simulink model "KF"  (R2019a)
settings: Solver=VariableStepAuto  StartTime=0.0  StopTime=200  RelTol=1e-3
values from neighbouring files (symbols this model uses):
  g = 9.81    [Q2.m]
  k_d_phi = (2*zeta_phi*omega_n_phi-a_phi_1)/a_phi_2    [Q2.m]
  k_i_chi = omega_n_chi^2*V_g/g    [Q2.m]
  k_i_phi = 0    [Q2.m]
  k_p_chi = 2*zeta_chi*omega_n_chi*V_g/g    [Q2.m]
  k_p_phi = delta_a_max/e_phi_max*sign(a_phi_2)    [Q2.m]
  V_g = 580/3.6    (= 161.111111111)    [Q2.m]
undefined symbols (not defined in the file or in its folder): sigbuilder_block
libraries: simulink_extras x3
settings Model: Creator=Shuyuan  LastModifiedBy=zhy
settings DataIOCC: ReturnWorkspaceOutputs=off
settings DebuggingCC: PregeneratedLibrarySubsystemCodeDiagnostic=none  ArithmeticOperatorsInVariantConditions=warning
settings SFSimCC: SimUseLocalCustomCode=off
settings RTWCC: RTWUseLocalCustomCode=off

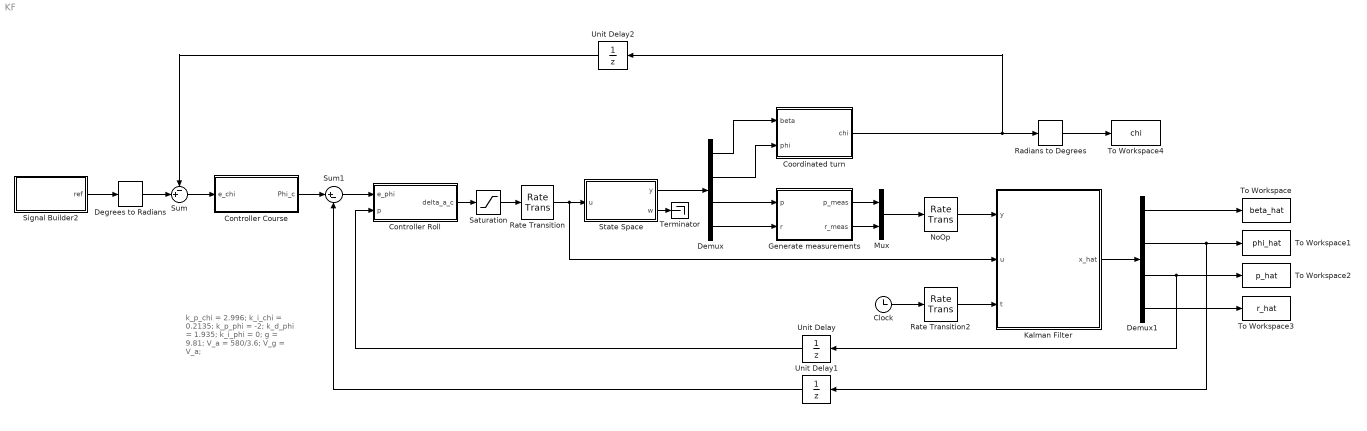
== system KF ==
  note: k_p_chi = 2.996;
      | k_i_chi = 0.2135;
      | k_p_phi = -2;
      | k_d_phi = 1.935;
      | k_i_phi = 0;
      |
      | g = 9.81;
      | V_a = 580/3.6;
      | V_g = V_a;
  Clock : Clock
  Controller Course : Subsystem
  Controller Roll : Subsystem
  Coordinated turn : Subsystem
  Degrees to Radians : simulink_extras/Transformations/Degrees to Radians
  Demux : Demux
  Demux1 : Demux
  Generate measurements : Subsystem
  Kalman Filter : MATLAB Function  TreatAsAtomicUnit=on
  Mux : Mux  Inputs=2
  NoOp : RateTransition
  Radians to Degrees : simulink_extras/Transformations/Radians to Degrees
  Rate Transition : RateTransition
  Rate Transition2 : RateTransition
  Saturation : Saturate  UpperLimit=30/180*pi  LowerLimit=-30/180*pi
  Signal Builder2 : Subsystem  Tag=STV Subsys  LoadFcn=sigbuilder_block('load');  StartFcn=sigbuilder_block('start');  StopFcn=sigbuilder_block('stop');  ClipboardFcn=sigbuilder_block('clipboard');  mask(Sigbuilder block){tuvar=[0:10]}
      mask help: Simulink:masks:SigbuilderBlock_MD
      mask init:
      | if ~strcmp(get_param(bdroot(gcbh),'SimulationStatus'),'stopped') tuvar = sigbuilder_block('maskInit'); end
      settings: CopyFcn=sigbuilder_block('copy');  DeleteFcn=sigbuilder_block('delete');  ModelCloseFcn=sigbuilder_block('modelClose');  PreSaveFcn=sigbuilder_block('preSave');  PauseFcn=sigbuilder_block('pause');  ContinueFcn=sigbuilder_block('continue');  NameChangeFcn=sigbuilder_block('namechange');  OpenFcn=sigbuilder_block('open',[411 163.2 550.8 400.2 ]);  CloseFcn=sigbuilder_block('close');
      mask Display: plot(0, 0, 100, 100,[2, 2, 32, 32, 2], [68, 8, 8, 68, 68],[32, 2], [38, 38], [32, 19, 2],[53, 60, 44], [32, 17, 17, 2],[16, 16, 31, 31]);txt = getActiveGroup(gcbh);text(2, 100, txt,'verticalAlignment', 'top');
  State Space : MATLAB Function  TreatAsAtomicUnit=on
  Sum : Sum  Inputs=-+|
  Sum1 : Sum  Inputs=|+-
  Terminator : Terminator
  To Workspace : ToWorkspace  VariableName=beta_hat  SaveFormat=Timeseries  SampleTime=-1
  To Workspace1 : ToWorkspace  VariableName=phi_hat  SaveFormat=Timeseries  SampleTime=-1
  To Workspace2 : ToWorkspace  VariableName=p_hat  SaveFormat=Timeseries  SampleTime=-1
  To Workspace3 : ToWorkspace  VariableName=r_hat  SaveFormat=Timeseries  SampleTime=-1
  To Workspace4 : ToWorkspace  VariableName=chi  SaveFormat=Timeseries  SampleTime=-1
  Unit Delay : UnitDelay  SampleTime=-1  HasFrameUpgradeWarning=on
  Unit Delay1 : UnitDelay  SampleTime=-1  HasFrameUpgradeWarning=on
  Unit Delay2 : UnitDelay  SampleTime=-1  HasFrameUpgradeWarning=on
  wires:
  Signal Builder2/1(ref) -> Degrees to Radians/1
  Sum/1 -> Controller Course/1(e_chi)
  Controller Course/1(Phi_c) -> Sum1/1
  Sum1/1 -> Controller Roll/1(e_phi)
  Controller Roll/1(delta_a_c) -> Saturation/1
  Rate Transition/1 -> Kalman Filter/2(u), State Space/1(u)
  State Space/1(y) -> Demux/1
  Demux/1 -> Coordinated turn/1(beta)
  Demux/2 -> Coordinated turn/2(phi)
  Demux/3 -> Generate measurements/1(p)
  Demux/4 -> Generate measurements/2(r)
  Clock/1 -> Rate Transition2/1
  Rate Transition2/1 -> Kalman Filter/3(t)
  Demux1/1 -> To Workspace/1
  Demux1/3 -> Unit Delay/1, To Workspace2/1
  Demux1/2 -> Unit Delay1/1, To Workspace1/1
  Demux1/4 -> To Workspace3/1
  Unit Delay/1 -> Controller Roll/2(p)
  Unit Delay1/1 -> Sum1/2
  State Space/2(w) -> Terminator/1
  Generate measurements/2(r_meas) -> Mux/2
  Generate measurements/1(p_meas) -> Mux/1
  Mux/1 -> NoOp/1
  NoOp/1 -> Kalman Filter/1(y)
  Kalman Filter/1(x_hat) -> Demux1/1
  Saturation/1 -> Rate Transition/1
  Radians to Degrees/1 -> To Workspace4/1
  Coordinated turn/1(chi) -> Unit Delay2/1, Radians to Degrees/1
  Degrees to Radians/1 -> Sum/2
  Unit Delay2/1 -> Sum/1

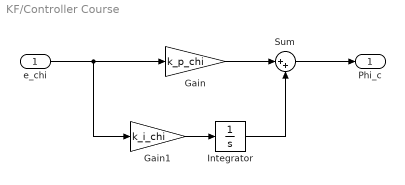
== system KF/Controller Course ==
  e_chi : Inport
  Gain : Gain  Gain=k_p_chi
  Gain1 : Gain  Gain=k_i_chi
  Integrator : Integrator
  Sum : Sum  Inputs=|++
  Phi_c : Outport
  wires:
  Sum/1 -> Phi_c/1
  Gain/1 -> Sum/1
  e_chi/1 -> Gain1/1, Gain/1
  Gain1/1 -> Integrator/1
  Integrator/1 -> Sum/2

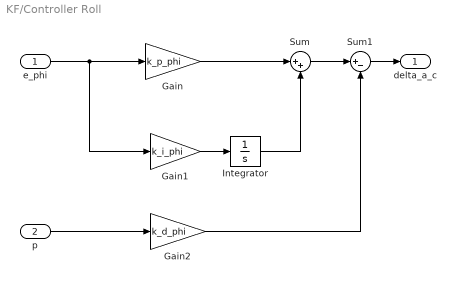
== system KF/Controller Roll ==
  e_phi : Inport
  p : Inport  Port=2
  Gain : Gain  Gain=k_p_phi
  Gain1 : Gain  Gain=k_i_phi
  Gain2 : Gain  Gain=k_d_phi
  Integrator : Integrator
  Sum : Sum  Inputs=|++
  Sum1 : Sum  Inputs=|+-
  delta_a_c : Outport
  wires:
  Gain/1 -> Sum/1
  e_phi/1 -> Gain1/1, Gain/1
  Gain1/1 -> Integrator/1
  Integrator/1 -> Sum/2
  Sum/1 -> Sum1/1
  Sum1/1 -> delta_a_c/1
  p/1 -> Gain2/1
  Gain2/1 -> Sum1/2

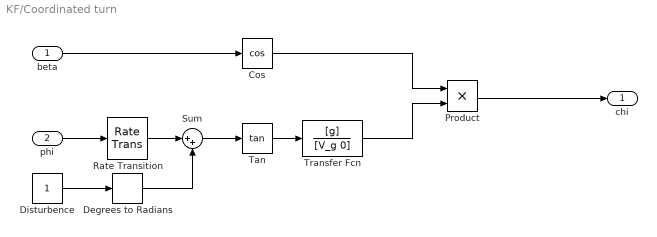
== system KF/Coordinated turn ==
  beta : Inport
  phi : Inport  Port=2
  Cos : Trigonometry  Operator=cos
  Degrees to Radians : simulink_extras/Transformations/Degrees to Radians
  Disturbence : Constant
  Product : Product
  Rate Transition : RateTransition
  Sum : Sum  Inputs=|++
  Tan : Trigonometry  Operator=tan
  Transfer Fcn : TransferFcn  Numerator=[g]  Denominator=[V_g 0]
  chi : Outport
  wires:
  phi/1 -> Rate Transition/1
  Disturbence/1 -> Degrees to Radians/1
  beta/1 -> Cos/1
  Sum/1 -> Tan/1
  Tan/1 -> Transfer Fcn/1
  Cos/1 -> Product/1
  Transfer Fcn/1 -> Product/2
  Degrees to Radians/1 -> Sum/2
  Rate Transition/1 -> Sum/1
  Product/1 -> chi/1

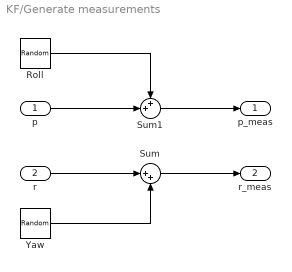
== system KF/Generate measurements ==
  p : Inport
  r : Inport  Port=2
  Roll : RandomNumber  Variance=(0.2*pi/180)^2  SampleTime=0.01
  Sum : Sum  Inputs=|++
  Sum1 : Sum  Inputs=++|
  Yaw : RandomNumber  Variance=(0.2*pi/180)^2  SampleTime=0.01
  p_meas : Outport
  r_meas : Outport  Port=2
  wires:
  p/1 -> Sum1/2
  Sum1/1 -> p_meas/1
  r/1 -> Sum/1
  Sum/1 -> r_meas/1
  Yaw/1 -> Sum/2
  Roll/1 -> Sum1/1

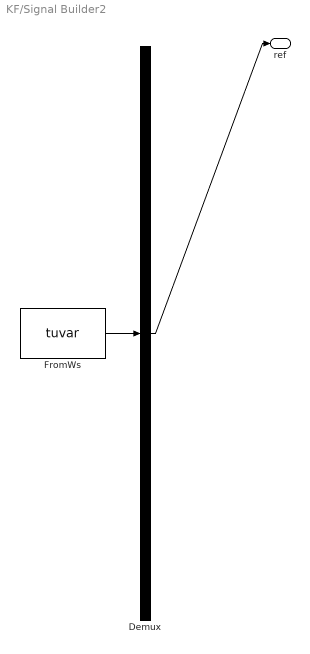
== system KF/Signal Builder2 ==
  Demux : Demux  Tag=STV Demux  Outputs=1
  FromWs : FromWorkspace  Tag=STV FromWs  VariableName=tuvar  SampleTime=0
      SigBuilderData=|
      | common.afterFinalStr = 'Extrapolate'
      | common.sampleTime = 0
      | dataSet.timeRange = [0 200]
      | dataSet.name = 'Group 1'
      | sbobj.Groups.Name = 'Group 1'
      | sbobj.Groups.Signals.Name = 'ref'
      | sbobj.Groups.Signals.XData = [0 25 25 75 75 125 125 200]
      | sbobj.Groups.Signals.YData = [0 0 5 5 10 10 15 15]
      | sbobj.Groups.TimeRange = [0 200]
  ref : Outport  Tag=STV Outport
  wires:
  FromWs/1 -> Demux/1
  Demux/1 -> ref/1

== matlab function KF/Kalman Filter ==
  settings: updateMethod=DISCRETE  sampleTime=0.01
  data: y input; x_hat output; u input; t input
function x_hat = Kalman_filter(y,u,t)

persistent xhat;
persistent xbar;
persistent P;

%% KF parameters
h = 0.01;
A_k = [-0.322, 0.052, 0.028, -1.12;
       0, 0, 1, -0.001;   
       -10.6, 0, -2.87, 0.46;
       6.87, 0, -0.04, -0.32];
B_k = [0.002; 0; -0.65; -0.02];
C_k = [0, 0, 1, 0;
       0, 0, 0, 1];
E_k = eye(4);
I = eye(4);
A_d = I+h*A_k;
B_d = h*B_k;
E_d = E_k;
Q = h*10^(-6)*diag([0.001,1,100,10]);
r = (0.2*pi/360)^2;
R = diag([r,r]);

%% Initial conditions
if isempty(xbar)
    xbar = [0;0;0;0];
    P = [0, 0, 0, 0;
         0, 0, 0, 0;
         0, 0, 0, 0;
         0, 0, 0, 0];
end

%% KF calculation
% if t <= 100
%     if mod(t, h) == 0
%     z = y;
%     H = C_k;
%     else
%     z = [0;0];
%     H = [0, 0, 0, 0; 0, 0, 0, 0];
%     end
% else
%     z = [0;0];
%     H = [0, 0, 0, 0; 0, 0, 0, 0];
% end


 if mod(t, h) == 0
    z = y;
    H = C_k;
 else
    z = [0;0];
    H = [0, 0, 0, 0; 0, 0, 0, 0];
 end



K = P*H'/(H*P*H'+R);
xhat = xbar+K*(z-H*xbar);
P = (I-K*H)*P*(I-K*H)'+K*R*K';

xbar = A_d*xhat+B_d*u;
P = A_d*P*A_d'+E_d*Q*E_d';

%% States output
x_hat = xhat;

== matlab function KF/State Space ==
  settings: updateMethod=DISCRETE  sampleTime=0.01
  data: u input; y output; w output
function [y,w] = state_space(u)
% Generate the output of the state space

    % Persistent variables to be kept between function calls
    persistent counter; % Variable for checking if it is the first iteration.
    persistent x;       % The state x
    
   % The next line is necessary for generating unique process noise for every simulation.
   % Otherwise, the noise will be equal every time you run the simulation,
   % even though it is white. This has to do with how Matlab generates
   % random numbers. 
   coder.extrinsic('randn','rng');
    
    h = 0.01;       % Time step of Euler integration
    delta_a_c = u;  % Aileron input
    
    if isempty(counter)
      % First iteration
        counter = 1;
           
        % Initialize state space
        x = zeros(5,1);
        w = zeros(5,1); 
        rng('shuffle'); % Necessary for generating unique process noise for every simulation.
    
    else
        % State-space matrices
        A = [-0.322, 0.052, 0.028, -1.12, 0.002;
             0, 0, 1, -0.001, 0;
             -10.6, 0, -2.87, 0.46, -0.65;
             6.87, 0, -0.04, -0.32, -0.02;
             0, 0, 0, 0, -7.5];
 
        B = [0; 0; 0; 0; 7.5;];
        
        E = eye(5);
        
        % Discrete version
        Ad = eye(5) + h*A;
        Bd = h*B;
        Ed = E;
        
        % The Qd matrix in the assignment is given directly in discrete-time here and
        % therefore, it is not necessary to discretize E.
        Qd = h*10^-6*[0.001, 0, 0, 0, 0;
                  0, 1, 0, 0, 0;
                  0, 0, 100, 0, 0;
                  0, 0, 0, 10, 0;
                  0, 0, 0, 0, 0];
          
        w = sqrt(Qd)*randn(5,1,1); % The standard deviation must be multiplied with random numbers with a zero-mean unit variance random number to generate process noise. 
        
        % Discrete-time state space update
        x = Ad*x + Bd * delta_a_c + Ed*w;
    end
    y = x(1:4); % Return every state except the actuator state.
end
